simulink model "Expt_3_2"  (R2018a)
settings: Solver=VariableStepAuto  StartTime=0.0  StopTime=10.0  RelTol=1e-3
settings Model: Creator=HP  LastModifiedBy=HP

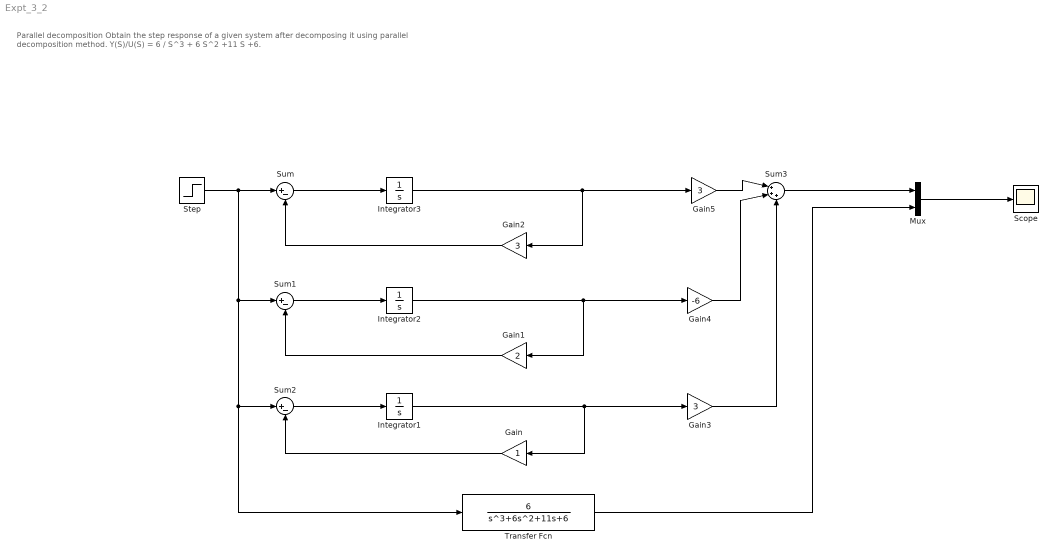
== system Expt_3_2 ==
  note: Parallel decomposition
      |
      | Obtain the step response of a given system after decomposing it using parallel decomposition method.
      |
      | Y(S)/U(S) = 6 / S^3 + 6 S^2 +11 S +6.
  Gain : Gain
  Gain1 : Gain  Gain=2
  Gain2 : Gain  Gain=3
  Gain3 : Gain  Gain=3
  Gain4 : Gain  Gain=-6
  Gain5 : Gain  Gain=3
  Integrator1 : Integrator
  Integrator2 : Integrator
  Integrator3 : Integrator
  Mux : Mux  Inputs=2
  Scope : Scope
  Step : Step  SampleTime=0
  Sum : Sum  Inputs=|+-
  Sum1 : Sum  Inputs=|+-
  Sum2 : Sum  Inputs=|+-
  Sum3 : Sum  Inputs=|+++
  Transfer Fcn : TransferFcn  Numerator=[6]  Denominator=[1 6 11 6]
  wires:
  Integrator3/1 -> Gain2/1, Gain5/1
  Integrator2/1 -> Gain1/1, Gain4/1
  Integrator1/1 -> Gain/1, Gain3/1
  Sum2/1 -> Integrator1/1
  Sum1/1 -> Integrator2/1
  Sum/1 -> Integrator3/1
  Step/1 -> Transfer Fcn/1, Sum2/1, Sum1/1, Sum/1
  Gain2/1 -> Sum/2
  Gain1/1 -> Sum1/2
  Gain/1 -> Sum2/2
  Transfer Fcn/1 -> Mux/2
  Gain5/1 -> Sum3/1
  Gain4/1 -> Sum3/2
  Gain3/1 -> Sum3/3
  Sum3/1 -> Mux/1
  Mux/1 -> Scope/1
